simulink model "Q17"  (Simulink 9.1)
settings: Solver=VariableStepAuto  StartTime=0.0  StopTime=10.0  RelTol=1e-3
settings Model: Creator=GamePC  LastModifiedBy=GamePC
settings DataIOCC: SaveFormat=Dataset
settings OptimizationCC: LifeSpan=auto
settings DebuggingCC: UnderspecifiedInitializationDetection=Simplified  MergeDetectMultiDrivingBlocksExec=error  SFUnexpectedBacktrackingDiag=error  SFNoUnconditionalDefaultTransitionDiag=error  SFExecutionAtInitializationDiag=warning
settings HardwareCC: ProdBitPerPointer=64  ProdBitPerSizeT=64  ProdBitPerPtrDiffT=64  ProdLargestAtomicFloat=Float  ProdIntDivRoundTo=Zero  ProdEndianess=LittleEndian  ProdWordSize=64  ProdHWDeviceType=Intel->x86-64 (Windows64)
settings ModelReferenceCC: PropagateSignalLabelsOutOfModel=on
settings CodeAppCC: StateflowObjectComments=off
settings GRTTargetCC: TargetLangStandard=C99 (ISO)  CombineOutputUpdateFcns=on  GRTInterface=off
settings ConfigComp: CovMetricSettings=dwe  CovHtmlReporting=off  CovSaveCumulativeToWorkspaceVar=off  CovSaveSingleToWorkspaceVar=off  CovExternalEMLEnable=on

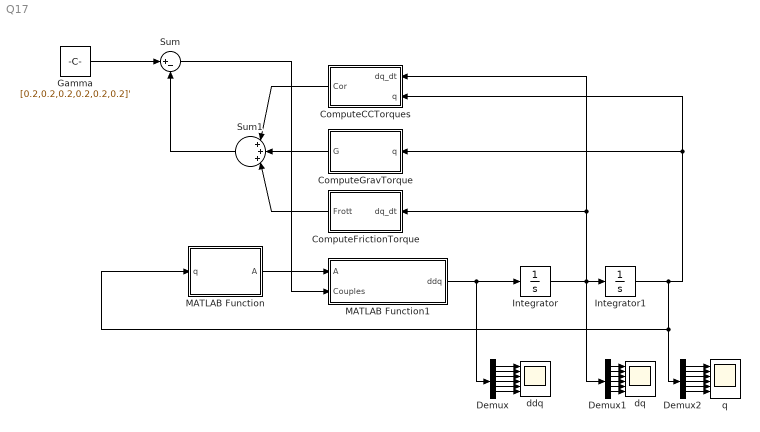
== system Q17 ==
  ComputeCCTorques : MATLAB Function  TreatAsAtomicUnit=on
  ComputeFrictionTorque : MATLAB Function  TreatAsAtomicUnit=on
  ComputeGravTorque : MATLAB Function  TreatAsAtomicUnit=on
  Demux : Demux  Outputs=6
  Demux1 : Demux  Outputs=6
  Demux2 : Demux  Outputs=6
  Gamma : Constant  Value=[0.2,0.2,0.2,0.2,0.2,0.2]'
  Integrator : Integrator
  Integrator1 : Integrator
  MATLAB Function : MATLAB Function  TreatAsAtomicUnit=on
  MATLAB Function1 : MATLAB Function  TreatAsAtomicUnit=on
  Sum : Sum  Inputs=|+-
  Sum1 : Sum  Inputs=|+++|
  "ddq " : Scope  NumInputPorts=6
  dq : Scope  NumInputPorts=6
  q : Scope  NumInputPorts=6
  wires:
  Integrator1/1 -> ComputeCCTorques/2(q), ComputeGravTorque/1(q), Demux2/1, MATLAB Function/1(q)
  Integrator/1 -> Demux1/1, ComputeCCTorques/1(dq_dt), ComputeFrictionTorque/1(dq_dt), Integrator1/1
  MATLAB Function1/1(ddq) -> Demux/1, Integrator/1
  MATLAB Function/1(A) -> MATLAB Function1/1(A)
  ComputeCCTorques/1(Cor) -> Sum1/1
  ComputeGravTorque/1(G) -> Sum1/2
  ComputeFrictionTorque/1(Frott) -> Sum1/3
  Sum1/1 -> Sum/2
  Sum/1 -> MATLAB Function1/2(Couples)
  Gamma/1 -> Sum/1
  Demux/1 -> "ddq "/1
  Demux/2 -> "ddq "/2
  Demux/3 -> "ddq "/3
  Demux/4 -> "ddq "/4
  Demux/5 -> "ddq "/5
  Demux/6 -> "ddq "/6
  Demux1/1 -> dq/1
  Demux1/2 -> dq/2
  Demux1/3 -> dq/3
  Demux1/4 -> dq/4
  Demux1/5 -> dq/5
  Demux1/6 -> dq/6
  Demux2/1 -> q/1
  Demux2/2 -> q/2
  Demux2/3 -> q/3
  Demux2/4 -> q/4
  Demux2/5 -> q/5
  Demux2/6 -> q/6

== matlab function MATLAB Function ==
  data: q input double; A output double
function A = ComputeMatInert(q)
    %set parameter
    m = [15,10,1,7,1,0.5];
    x_G1 = 0; y_G1 = 0; z_G1 = -0.25;
    x_G2 = 0.35; y_G2 = 0; z_G2 = 0;
    x_G3 = 0; y_G3 = -0.1; z_G3 = 0;
    x_G4 = 0; y_G4 = 0; z_G4 = 0;
    x_G5 = 0; y_G5 = 0; z_G5 = 0;
    x_G6 = 0; y_G6 = 0; z_G6 = 0;
    x_G=[x_G1 x_G2 x_G3 x_G4 x_G5 x_G6]';
    y_G=[y_G1 y_G2 y_G3 y_G4 y_G5 y_G6]';
    z_G=[z_G1 z_G2 z_G3 z_G4 z_G5 z_G6]';
    
    iI = zeros(3,3,6);
    iI(:,:,1)=[0.80 0 0.05 ; 0 0.80 0 ; 0.05  0  0.10];
    iI(:,:,2)=[0.10  0  0.10; 0  1.50 0 ; 0.10  0  1.50];
    iI(:,:,3)=[0.05 0 0 ; 0 0.01 0 ; 0 0 0.05];
    iI(:,:,4)=[0.50 0 0 ; 0 0.50 0 ; 0 0 0.05];
    iI(:,:,5)=[0.01 0 0 ; 0 0.01 0 ; 0 0 0.01];
    iI(:,:,6)=[0.01 0 0 ; 0 0.01 0 ; 0 0 0.01];
    
    d3 = 0.7; d = [0,0,d3,0,0,0];
    r1 = 0.5; r4 = 0.2; r = [r1,0,0,r4,0,0];   
    alpha = [ 0 , pi/2 , 0 , pi/2 , -pi/2 , pi/2 ];
    theta = zeros(6,1);
    theta = [q(1) q(2) q(3)+pi/2 q(4) q(5) q(6)]';
    Rred = [100 100 100 70 70 70];
    Jm = 1e-5*[1 1 1 1 1 1];
    %initialization of result
    %A = zeros(size(q,1),size(q,1));
    A = zeros(6,6);
    
    g_0i = eye(4);
    g_elem = eye(4);
    OJv_Gi = zeros(3,6);
    OJ_wi = zeros(3,6);
    [OJv_Gi,OJ_wi] = CalculMatriceJacobienneGi(alpha, d, theta, r, x_G, y_G, z_G);
    
    for i = 1:length(q)
        OPreproduitVect_OiGi = [0, -z_G(i), y_G(i);z_G(i),0,-x_G(i);-y_G(i),x_G(i),0];
        %mH = m(i)*OPreproduitVect_OiGi*OPreproduitVect_OiGi
        iI_Gi = iI(:,:,i)+m(i)*OPreproduitVect_OiGi*OPreproduitVect_OiGi;
        
        g_elem = TransformMatElem(alpha(i),d(i),theta(i),r(i));
        g_0i = g_0i*g_elem;
        ROi = g_0i(1:3,1:3);
        
        %OI_Gi = ROi(:,:,i)*iI_Gi*ROi(:,:,i)';
        OI_Gi = ROi*iI_Gi*ROi';
        A = A + (m(i)*OJv_Gi(:,:,i)')*OJv_Gi(:,:,i)+(OJ_wi(:,:,i)')*OI_Gi*OJ_wi(:,:,i);       
    end
A = A + diag(Rred.^2.*Jm);
end

== matlab function ComputeCCTorques ==
  data: dq_dt input double; q input double; Cor output double size=[6,1]
function Cor = fcn(dq_dt, q)
    Cor = zeros(6,1);
    Cor =ComputeCCTorques(q,dq_dt)'; 

end

== matlab function MATLAB Function1 ==
  data: A input double; ddq output double size=6; Couples input double
function ddq = fcn(A, Couples)

ddq = A\Couples;
end

== matlab function ComputeGravTorque ==
  data: q input double; G output double size=6
function G = fcn(q)
    
    G = ComputeGravTorque(q);

end

== matlab function ComputeFrictionTorque ==
  data: dq_dt input double; Frott output double size=6
function Frott = ComputFrictionTorque(dq_dt)
    %parametres
    Fv = 10*ones(6,1);
    
    %Fonction donnée à l'interieure du TP
    Frott = diag(dq_dt)*Fv;
   
end
